simulink model "st_transient"  (R2025b)
settings: Solver=VariableStepAuto  StartTime=0.0  StopTime=t_sim  RelTol=1e-3
values from neighbouring files (symbols this model uses):
  A_oins = 0.6*pi*r3    [st_transient_parameters.m]
  mcp_IT3 = m_air*cp_air    (= 318.000965941)    [st_transient_parameters.m]
  mcp_RP1 = m_RP1*cp_RP1 + m_wall*cp_al    (= 61.4260182409)    [st_transient_parameters.m]
  R_ins = 0    [st_transient_parameters.m]
  T_inf = 270    [st_transient_parameters.m]
  T_IT3_i = 290    [st_transient_parameters.m]
  T_lox = 90    [st_transient_parameters.m]
  T_RP1_i = 290    [st_transient_parameters.m]
settings Model: Creator=aryan  LastModifiedBy=aryan

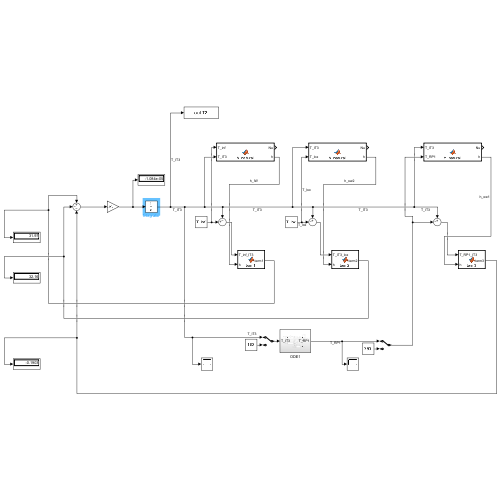
[thumbnail: Simulink's stored preview of the top-level diagram]
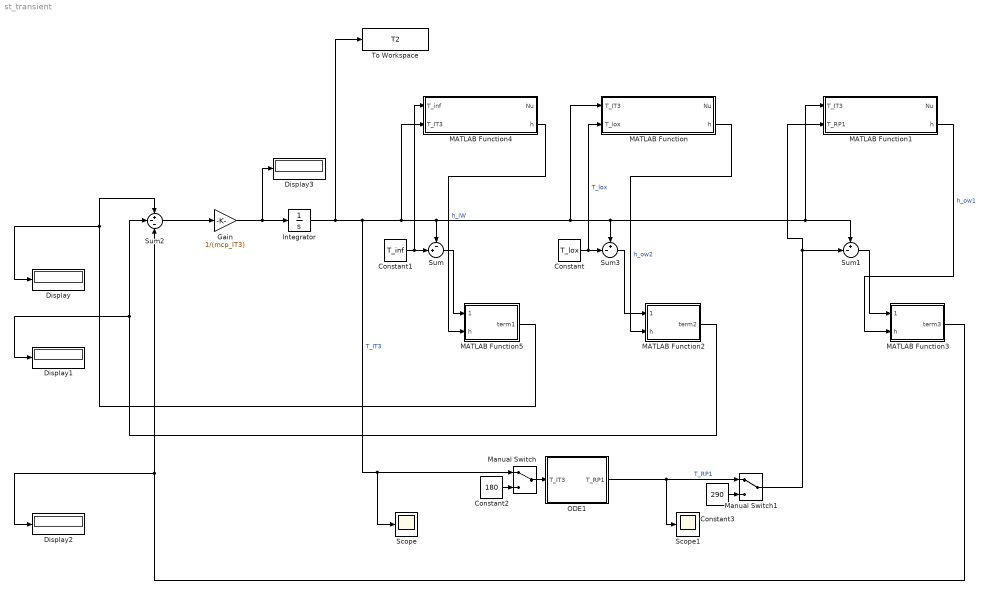
== system st_transient ==
  Constant : Constant  Value=T_lox
  Constant1 : Constant  Value=T_inf
  Constant2 : Constant  Value=180
  Constant3 : Constant  Value=290
  Display{,1..3} (4 alike) : Display
  Gain : Gain  Gain=1/(mcp_IT3)
  Integrator : Integrator  InitialCondition=T_IT3_i
  MATLAB Function : MATLAB Function  TreatAsAtomicUnit=on
  MATLAB Function1 : MATLAB Function  TreatAsAtomicUnit=on
  MATLAB Function2 : MATLAB Function  TreatAsAtomicUnit=on
  MATLAB Function3 : MATLAB Function  TreatAsAtomicUnit=on
  MATLAB Function4 : MATLAB Function  TreatAsAtomicUnit=on
  MATLAB Function5 : MATLAB Function  TreatAsAtomicUnit=on
  Manual Switch : ManualSwitch
  Manual Switch1 : ManualSwitch
  ODE1 : Subsystem
  Scope : Scope
      settings: ActiveDisplayYMinimum=20454.125262270652  ActiveDisplayYMaximum=85234.910913952568  DataLoggingVariableName=ScopeData4
  Scope1 : Scope
      settings: ActiveDisplayYMinimum=-2.6364014505129E+83  ActiveDisplayYMaximum=1.7393776682186235E+84  DataLoggingVariableName=ScopeData5
  Sum : Sum  Inputs=-+|
  Sum1 : Sum  Inputs=+-|
  Sum2 : Sum  Inputs=+--
  Sum3 : Sum  Inputs=+-|
  To Workspace : ToWorkspace  VariableName=T2  SaveFormat=Timeseries  SampleTime=-1
  wires:
  Integrator/1 -> To Workspace/1, MATLAB Function4/2(T_IT3), MATLAB Function/1(T_IT3), Sum1/1, MATLAB Function1/1(T_IT3), Sum3/1, Sum/1, Manual Switch/1, Scope/1  "T_IT3"
  ODE1/1(T_RP1) -> Scope1/1, Manual Switch1/1  "T_RP1"
  Constant1/1 -> MATLAB Function4/1(T_inf), Sum/2
  Constant/1 -> MATLAB Function/2(T_lox), Sum3/2  "T_lox"
  Gain/1 -> Display3/1, Integrator/1
  Sum2/1 -> Gain/1
  MATLAB Function3/1(term3) -> Display2/1, Sum2/3
  MATLAB Function5/1(term1) -> Display/1, Sum2/1
  MATLAB Function2/1(term2) -> Display1/1, Sum2/2
  MATLAB Function/2(h) -> MATLAB Function2/2(h)  "h_ow2"
  Sum3/1 -> MATLAB Function2/1(T_IT3_lox)
  MATLAB Function1/2(h) -> MATLAB Function3/2(h)  "h_ow1"
  Sum1/1 -> MATLAB Function3/1(T_RP1_IT3)
  MATLAB Function4/2(h) -> MATLAB Function5/2(h)  "h_iW"
  Sum/1 -> MATLAB Function5/1(T_inf_IT3)
  Manual Switch/1 -> ODE1/1(T_IT3)
  Constant2/1 -> Manual Switch/2
  Manual Switch1/1 -> MATLAB Function1/2(T_RP1), Sum1/2
  Constant3/1 -> Manual Switch1/2

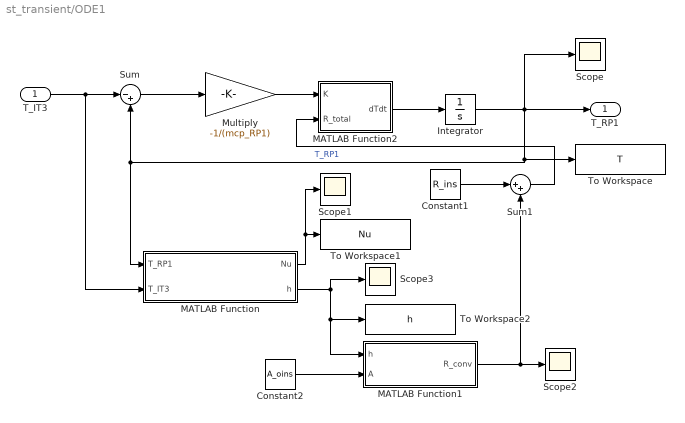
== system st_transient/ODE1 ==
  T_IT3 : Inport
  Constant1 : Constant  Value=R_ins
  Constant2 : Constant  Value=A_oins
  Integrator : Integrator  InitialCondition=T_RP1_i
  MATLAB Function : MATLAB Function  TreatAsAtomicUnit=on
  MATLAB Function1 : MATLAB Function  TreatAsAtomicUnit=on
  MATLAB Function2 : MATLAB Function  TreatAsAtomicUnit=on
  Multiply : Gain  Gain=-1/(mcp_RP1)
  Scope{,1..3} (4 alike) : Scope
      Scope settings: ActiveDisplayYMinimum=260.25246238308375  ActiveDisplayYMaximum=321.33069422822069
      Scope1 settings: ActiveDisplayYMinimum=-1  ActiveDisplayYMaximum=1
      Scope2 settings: ActiveDisplayYMinimum=-31.29088337884123  ActiveDisplayYMaximum=45.896592661263512  DataLoggingVariableName=ScopeData2
      Scope3 settings: ActiveDisplayYMinimum=-1.453026566225704  ActiveDisplayYMaximum=14.066469860499284  DataLoggingVariableName=ScopeData3
  Sum : Sum  Inputs=|-+
  Sum1 : Sum  Inputs=|++
  To Workspace : ToWorkspace  VariableName=T  SaveFormat=Timeseries  SampleTime=-1
  To Workspace1 : ToWorkspace  VariableName=Nu  SaveFormat=Timeseries  SampleTime=-1
  To Workspace2 : ToWorkspace  VariableName=h  SaveFormat=Timeseries  SampleTime=-1
  T_RP1 : Outport
  wires:
  Integrator/1 -> T_RP1/1, MATLAB Function/1(T_RP1), Sum/2, To Workspace/1, Scope/1  "T_RP1"
  T_IT3/1 -> MATLAB Function/2(T_IT3), Sum/1
  MATLAB Function2/1(dTdt) -> Integrator/1
  Multiply/1 -> MATLAB Function2/1(K)
  MATLAB Function/2(h) -> Scope3/1, To Workspace2/1, MATLAB Function1/1(h)
  Constant1/1 -> Sum1/1
  Constant2/1 -> MATLAB Function1/2(A)
  Sum/1 -> Multiply/1
  Sum1/1 -> MATLAB Function2/2(R_total)
  MATLAB Function/1(Nu) -> To Workspace1/1, Scope1/1
  MATLAB Function1/1(R_conv) -> Sum1/2, Scope2/1

== matlab function st_transient/ODE1/MATLAB Function1 ==
  data: h input; R_conv output; A input
function R_conv = Rconv(h, A)

    R_conv = 1/(h*A);

== matlab function st_transient/ODE1/MATLAB Function ==
  data: Nu output; h output; T_RP1 input; T_IT3 input
function [Nu, h] = h_natural(T_RP1, T_IT3)
    coder.extrinsic('getNusselt_natural')
    Nu = 0;
    h = 0;

    geo = 'vertical_plate';
    rho = 1.225;    % {kg/m^3}              T = 290 K, P within [0.5, 40] MPa
    mu = 0.001;     % {Pa*s}                T = 293 K
    k = 0.135;      % {W/m*K}
    cp = 1005;      % {J/kg*K}
    L = 0.127;      % {m}
    D = 0;          % {m} not needed for case: 'vertical_plate'
    
    % T_film = (T_IT3 + T_i)/2
    [Nu, h] = getNusselt_natural(geo, rho, mu, k, cp, L, D, T_RP1, T_IT3);

== matlab function st_transient/ODE1/MATLAB Function2 ==
  data: K input; R_total input; dTdt output
function dTdt = fcn(K, R_total)
    
    dTdt = K/R_total;

== matlab function st_transient/MATLAB Function ==
  data: T_IT3 input; Nu output; h output; T_lox input
function [Nu, h] = h_natural(T_IT3, T_lox)
    coder.extrinsic('getNusselt_natural')
    Nu = 0;
    h = 0;

    geo = 'vertical_plate';
    rho = 1.225;    % {kg/m^3}              T = 290 K, P within [0.5, 40] MPa
    mu = 0.001;     % {Pa*s}                T = 293 K
    k = 0.135;      % {W/m*K}
    cp = 1005;      % {J/kg*K}
    L = 0.127;      % {m}
    D = 0;          % {m} not needed for case: 'vertical_plate'
    
    % T_film = (T_IT3 + T_i)/2
    [Nu, h] = getNusselt_natural(geo, rho, mu, k, cp, L, D, T_lox, T_IT3);

== matlab function st_transient/MATLAB Function1 ==
  data: T_IT3 input; Nu output; h output; T_RP1 input
function [Nu, h] = h_natural(T_IT3, T_RP1)
    coder.extrinsic('getNusselt_natural')
    Nu = 0;
    h = 0;

    geo = 'vertical_plate';
    rho = 1.225;    % {kg/m^3}              T = 290 K, P within [0.5, 40] MPa
    mu = 0.001;     % {Pa*s}                T = 293 K
    k = 0.135;      % {W/m*K}
    cp = 1005;      % {J/kg*K}
    L = 0.127;      % {m}
    D = 0;          % {m} not needed for case: 'vertical_plate'
    
    % T_film = (T_IT3 + T_i)/2
    [Nu, h] = getNusselt_natural(geo, rho, mu, k, cp, L, D, T_RP1, T_IT3);

== matlab function st_transient/MATLAB Function2 ==
  data: T_IT3_lox input; term2 output; h input
function term2 = term2(T_IT3_lox, h)

    A_ow2 = 0.0233;
    R_iw2 = 1.7967;
    R_w2 = 1.7989e-04;
    R_ow2 = 1/(h*A_ow2);

    R_total = R_ow2 + R_w2 + R_iw2;

    term2 = T_IT3_lox/R_total;

== matlab function st_transient/MATLAB Function3 ==
  data: T_RP1_IT3 input; term3 output; h input
function term3 = term3(T_RP1_IT3, h)

    A_ow1 = 0.0075;
    R_iw1 = 4.2349;
    R_w1 = 5.2417e-05;
    R_ow1 = 1/(h*A_ow1);

    R_total = R_ow1 + R_w1 + R_iw1;

    term3 = T_RP1_IT3/R_total;

== matlab function st_transient/MATLAB Function4 ==
  data: T_inf input; T_IT3 input; Nu output; h output
function [Nu, h] = h_natural(T_inf, T_IT3)
    coder.extrinsic('getNusselt_natural')
    Nu = 0;
    h = 0;

    geo = 'vertical_plate';
    rho = 1.225;    % {kg/m^3}              T = 290 K, P within [0.5, 40] MPa
    mu = 0.001;     % {Pa*s}                T = 293 K
    k = 0.135;      % {W/m*K}
    cp = 1005;      % {J/kg*K}
    L = 0.127;      % {m}
    D = 0;          % {m} not needed for case: 'vertical_plate'
    
    % T_film = (T_IT3 + T_i)/2
    [Nu, h] = getNusselt_natural(geo, rho, mu, k, cp, L, D, T_IT3, T_inf);

== matlab function st_transient/MATLAB Function5 ==
  data: T_inf_IT3 input; term1 output; h input
function term1 = term1(T_inf_IT3, h)

    A_iW = 1.0242;
    R_oW = 0.0130;
    R_W = 0.0061;
    R_iW = 1/(h*A_iW);

    R_total = R_oW + R_W + R_iW;

    term1 = T_inf_IT3/R_total;
